simulink model "Hardware_Interface"  (R2021b)
settings: Solver=VariableStepAuto  StartTime=0.0  StopTime=10.0  RelTol=1e-3
settings Model: Creator=Natmatee  LastModifiedBy=Natmatee

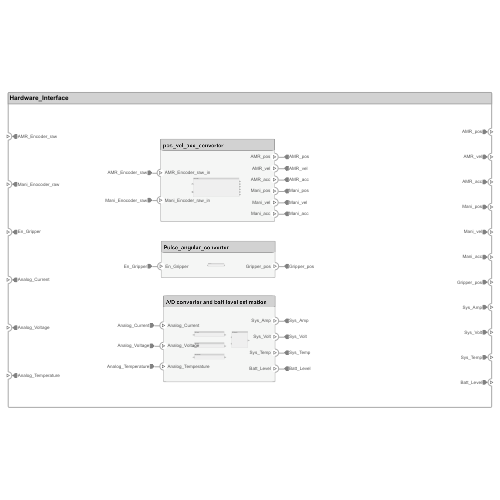
[thumbnail: Simulink's stored preview of the top-level diagram]
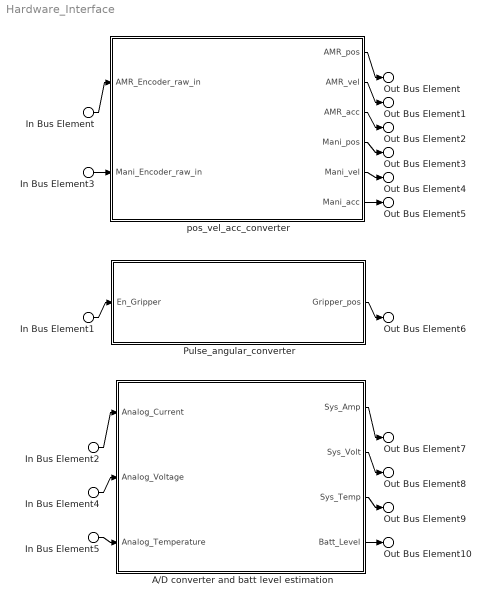
== system Hardware_Interface ==
  In Bus Element : Inport  PortName=AMR_Encoder_raw
  In Bus Element3 : Inport  Port=2  PortName=Mani_Enocoder_raw
  In Bus Element1 : Inport  Port=3  PortName=En_Gripper
  In Bus Element2 : Inport  Port=4  PortName=Analog_Current
  In Bus Element4 : Inport  Port=5  PortName=Analog_Voltage
  In Bus Element5 : Inport  Port=6  PortName=Analog_Temperature
  A/D converter and batt level estimation : Subsystem
      settings: PortSchema="{\"entries\":[{\"content\":{\"headerSize\":26,\"margin\":15,\"minimumSpacing\":25,\"sides\":[{\"content\":{\"connectorIds\":[\"In1\",\"In2\",\"In3\"]},\"type\":\"ConnectorPlacement.EquallySpacedRectSide\",\"uuid\":\"981ec522-52a0-4dbf-ac20-b0bdc6aa1afd\"},{\"content\":{\"connectorIds\":[\"Out1\",\"Out2\",\"Out3\",\"Out4\"],\"side\":\"RIGHT\"},\"type\":\"ConnectorPlacement.EquallySpacedRectSide\",\"uuid\":\"9bffbeba-24b3-4025-8564-8c4b0e924e04\"},{\"content\":{\"connectorIds\":[],\"side\":\"TOP\"},\"type\":\"ConnectorPlacement.EquallySpacedRectSide\",\"uuid\":\"d6517fca-b776-44cd-80b5-050d73676340\"}]},\"type\":\"ConnectorPlacement.EquallySpacedConnector\",\"uuid\":\"152addaa-b2c5-4af4-bfc3-3d7a632ca387\"}],\"packageUris\":[\"http://schema.mathworks.com/mf0/Connector/R2020b\"],\"version\":\"1.0\"}"
  Pulse_angular_converter : Subsystem
      settings: PortSchema="{\"entries\":[{\"content\":{\"headerSize\":26,\"margin\":15,\"minimumSpacing\":25,\"sides\":[{\"content\":{\"connectorIds\":[\"In1\"]},\"type\":\"ConnectorPlacement.EquallySpacedRectSide\",\"uuid\":\"981ec522-52a0-4dbf-ac20-b0bdc6aa1afd\"},{\"content\":{\"connectorIds\":[\"Out1\"],\"side\":\"RIGHT\"},\"type\":\"ConnectorPlacement.EquallySpacedRectSide\",\"uuid\":\"9bffbeba-24b3-4025-8564-8c4b0e924e04\"},{\"content\":{\"connectorIds\":[],\"side\":\"TOP\"},\"type\":\"ConnectorPlacement.EquallySpacedRectSide\",\"uuid\":\"d6517fca-b776-44cd-80b5-050d73676340\"}]},\"type\":\"ConnectorPlacement.EquallySpacedConnector\",\"uuid\":\"152addaa-b2c5-4af4-bfc3-3d7a632ca387\"}],\"packageUris\":[\"http://schema.mathworks.com/mf0/Connector/R2020b\"],\"version\":\"1.0\"}"
  pos_vel_acc_converter : Subsystem
      settings: PortSchema="{\"entries\":[{\"content\":{\"headerSize\":26,\"margin\":15,\"minimumSpacing\":25,\"sides\":[{\"content\":{\"connectorIds\":[\"In1\",\"In2\"]},\"type\":\"ConnectorPlacement.EquallySpacedRectSide\",\"uuid\":\"981ec522-52a0-4dbf-ac20-b0bdc6aa1afd\"},{\"content\":{\"connectorIds\":[\"Out1\",\"Out2\",\"Out3\",\"Out4\",\"Out5\",\"Out6\"],\"side\":\"RIGHT\"},\"type\":\"ConnectorPlacement.EquallySpacedRectSide\",\"uuid\":\"9bffbeba-24b3-4025-8564-8c4b0e924e04\"},{\"content\":{\"connectorIds\":[],\"side\":\"TOP\"},\"type\":\"ConnectorPlacement.EquallySpacedRectSide\",\"uuid\":\"d6517fca-b776-44cd-80b5-050d73676340\"}]},\"type\":\"ConnectorPlacement.EquallySpacedConnector\",\"uuid\":\"152addaa-b2c5-4af4-bfc3-3d7a632ca387\"}],\"packageUris\":[\"http://schema.mathworks.com/mf0/Connector/R2020b\"],\"version\":\"1.0\"}"
  Out Bus Element : Outport  PortName=AMR_pos
  Out Bus Element1 : Outport  Port=2  PortName=AMR_vel
  Out Bus Element2 : Outport  Port=3  PortName=AMR_acc
  Out Bus Element3 : Outport  Port=4  PortName=Mani_pos
  Out Bus Element4 : Outport  Port=5  PortName=Mani_vel
  Out Bus Element5 : Outport  Port=6  PortName=Mani_acc
  Out Bus Element6 : Outport  Port=7  PortName=Gripper_pos
  Out Bus Element7 : Outport  Port=8  PortName=Sys_Amp
  Out Bus Element8 : Outport  Port=9  PortName=Sys_Volt
  Out Bus Element9 : Outport  Port=10  PortName=Sys_Temp
  Out Bus Element10 : Outport  Port=11  PortName=Batt_Level
  wires:
  pos_vel_acc_converter/1(AMR_pos) -> Out Bus Element/1
  pos_vel_acc_converter/2(AMR_vel) -> Out Bus Element1/1
  pos_vel_acc_converter/3(AMR_acc) -> Out Bus Element2/1
  pos_vel_acc_converter/4(Mani_pos) -> Out Bus Element3/1
  pos_vel_acc_converter/5(Mani_vel) -> Out Bus Element4/1
  pos_vel_acc_converter/6(Mani_acc) -> Out Bus Element5/1
  In Bus Element2/1 -> A/D converter and batt level estimation/1(Analog_Current)
  In Bus Element4/1 -> A/D converter and batt level estimation/2(Analog_Voltage)
  In Bus Element5/1 -> A/D converter and batt level estimation/3(Analog_Temperature)
  A/D converter and batt level estimation/1(Sys_Amp) -> Out Bus Element7/1
  A/D converter and batt level estimation/2(Sys_Volt) -> Out Bus Element8/1
  A/D converter and batt level estimation/3(Sys_Temp) -> Out Bus Element9/1
  A/D converter and batt level estimation/4(Batt_Level) -> Out Bus Element10/1
  In Bus Element1/1 -> Pulse_angular_converter/1(En_Gripper)
  Pulse_angular_converter/1(Gripper_pos) -> Out Bus Element6/1
  In Bus Element/1 -> pos_vel_acc_converter/1(AMR_Encoder_raw_in)
  In Bus Element3/1 -> pos_vel_acc_converter/2(Mani_Encoder_raw_in)

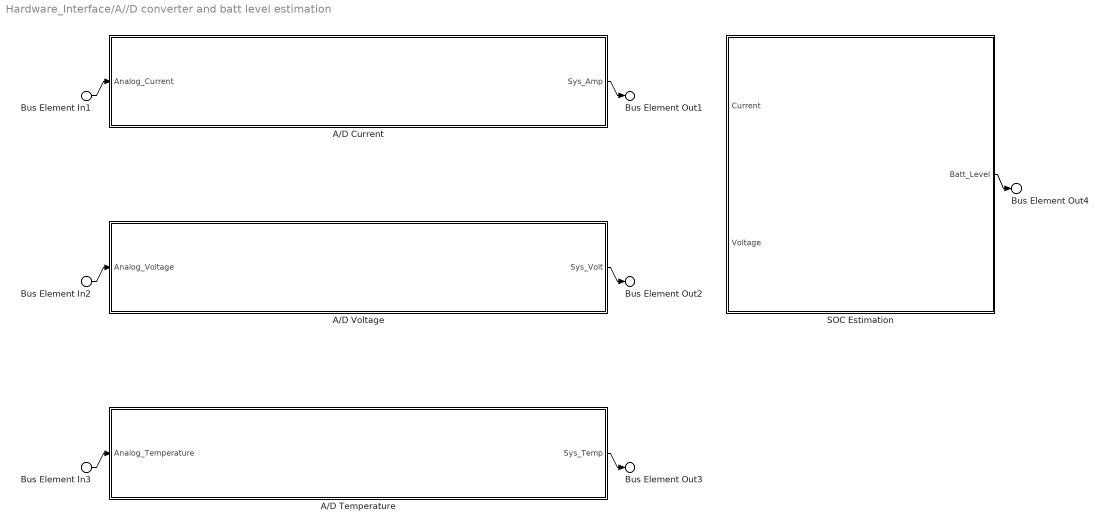
== system Hardware_Interface/A//D converter and batt level estimation ==
  Bus Element In1 : Inport  PortName=Analog_Current
  Bus Element In2 : Inport  Port=2  PortName=Analog_Voltage
  Bus Element In3 : Inport  Port=3  PortName=Analog_Temperature
  A/D Current : Subsystem
      settings: PortSchema="{\"entries\":[{\"content\":{\"headerSize\":26,\"margin\":15,\"minimumSpacing\":25,\"sides\":[{\"content\":{\"connectorIds\":[\"In1\"]},\"type\":\"ConnectorPlacement.EquallySpacedRectSide\",\"uuid\":\"981ec522-52a0-4dbf-ac20-b0bdc6aa1afd\"},{\"content\":{\"connectorIds\":[\"Out1\"],\"side\":\"RIGHT\"},\"type\":\"ConnectorPlacement.EquallySpacedRectSide\",\"uuid\":\"9bffbeba-24b3-4025-8564-8c4b0e924e04\"},{\"content\":{\"connectorIds\":[],\"side\":\"TOP\"},\"type\":\"ConnectorPlacement.EquallySpacedRectSide\",\"uuid\":\"d6517fca-b776-44cd-80b5-050d73676340\"}]},\"type\":\"ConnectorPlacement.EquallySpacedConnector\",\"uuid\":\"152addaa-b2c5-4af4-bfc3-3d7a632ca387\"}],\"packageUris\":[\"http://schema.mathworks.com/mf0/Connector/R2020b\"],\"version\":\"1.0\"}"
  A/D Temperature : Subsystem
      settings: PortSchema="{\"entries\":[{\"content\":{\"headerSize\":26,\"margin\":15,\"minimumSpacing\":25,\"sides\":[{\"content\":{\"connectorIds\":[\"In1\"]},\"type\":\"ConnectorPlacement.EquallySpacedRectSide\",\"uuid\":\"981ec522-52a0-4dbf-ac20-b0bdc6aa1afd\"},{\"content\":{\"connectorIds\":[\"Out1\"],\"side\":\"RIGHT\"},\"type\":\"ConnectorPlacement.EquallySpacedRectSide\",\"uuid\":\"9bffbeba-24b3-4025-8564-8c4b0e924e04\"},{\"content\":{\"connectorIds\":[],\"side\":\"TOP\"},\"type\":\"ConnectorPlacement.EquallySpacedRectSide\",\"uuid\":\"d6517fca-b776-44cd-80b5-050d73676340\"}]},\"type\":\"ConnectorPlacement.EquallySpacedConnector\",\"uuid\":\"152addaa-b2c5-4af4-bfc3-3d7a632ca387\"}],\"packageUris\":[\"http://schema.mathworks.com/mf0/Connector/R2020b\"],\"version\":\"1.0\"}"
  A/D Voltage : Subsystem
      settings: PortSchema="{\"entries\":[{\"content\":{\"headerSize\":26,\"margin\":15,\"minimumSpacing\":25,\"sides\":[{\"content\":{\"connectorIds\":[\"In1\"]},\"type\":\"ConnectorPlacement.EquallySpacedRectSide\",\"uuid\":\"981ec522-52a0-4dbf-ac20-b0bdc6aa1afd\"},{\"content\":{\"connectorIds\":[\"Out1\"],\"side\":\"RIGHT\"},\"type\":\"ConnectorPlacement.EquallySpacedRectSide\",\"uuid\":\"9bffbeba-24b3-4025-8564-8c4b0e924e04\"},{\"content\":{\"connectorIds\":[],\"side\":\"TOP\"},\"type\":\"ConnectorPlacement.EquallySpacedRectSide\",\"uuid\":\"d6517fca-b776-44cd-80b5-050d73676340\"}]},\"type\":\"ConnectorPlacement.EquallySpacedConnector\",\"uuid\":\"152addaa-b2c5-4af4-bfc3-3d7a632ca387\"}],\"packageUris\":[\"http://schema.mathworks.com/mf0/Connector/R2020b\"],\"version\":\"1.0\"}"
  SOC Estimation : Subsystem
      settings: PortSchema="{\"entries\":[{\"content\":{\"headerSize\":26,\"margin\":15,\"minimumSpacing\":25,\"sides\":[{\"content\":{\"connectorIds\":[\"In1\",\"In2\"]},\"type\":\"ConnectorPlacement.EquallySpacedRectSide\",\"uuid\":\"981ec522-52a0-4dbf-ac20-b0bdc6aa1afd\"},{\"content\":{\"connectorIds\":[\"Out1\"],\"side\":\"RIGHT\"},\"type\":\"ConnectorPlacement.EquallySpacedRectSide\",\"uuid\":\"9bffbeba-24b3-4025-8564-8c4b0e924e04\"},{\"content\":{\"connectorIds\":[],\"side\":\"TOP\"},\"type\":\"ConnectorPlacement.EquallySpacedRectSide\",\"uuid\":\"d6517fca-b776-44cd-80b5-050d73676340\"}]},\"type\":\"ConnectorPlacement.EquallySpacedConnector\",\"uuid\":\"152addaa-b2c5-4af4-bfc3-3d7a632ca387\"}],\"packageUris\":[\"http://schema.mathworks.com/mf0/Connector/R2020b\"],\"version\":\"1.0\"}"
  Bus Element Out1 : Outport  PortName=Sys_Amp
  Bus Element Out2 : Outport  Port=2  PortName=Sys_Volt
  Bus Element Out3 : Outport  Port=3  PortName=Sys_Temp
  Bus Element Out4 : Outport  Port=4  PortName=Batt_Level
  wires:
  A/D Current/1(Sys_Amp) -> Bus Element Out1/1
  Bus Element In1/1 -> A/D Current/1(Analog_Current)
  A/D Voltage/1(Sys_Volt) -> Bus Element Out2/1
  Bus Element In2/1 -> A/D Voltage/1(Analog_Voltage)
  Bus Element In3/1 -> A/D Temperature/1(Analog_Temperature)
  A/D Temperature/1(Sys_Temp) -> Bus Element Out3/1
  SOC Estimation/1(Batt_Level) -> Bus Element Out4/1

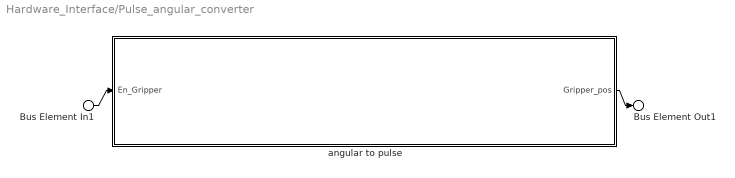
== system Hardware_Interface/Pulse_angular_converter ==
  Bus Element In1 : Inport  PortName=En_Gripper
  angular to pulse : Subsystem
      settings: PortSchema="{\"entries\":[{\"content\":{\"headerSize\":26,\"margin\":15,\"minimumSpacing\":25,\"sides\":[{\"content\":{\"connectorIds\":[\"In1\"]},\"type\":\"ConnectorPlacement.EquallySpacedRectSide\",\"uuid\":\"981ec522-52a0-4dbf-ac20-b0bdc6aa1afd\"},{\"content\":{\"connectorIds\":[\"Out1\"],\"side\":\"RIGHT\"},\"type\":\"ConnectorPlacement.EquallySpacedRectSide\",\"uuid\":\"9bffbeba-24b3-4025-8564-8c4b0e924e04\"},{\"content\":{\"connectorIds\":[],\"side\":\"TOP\"},\"type\":\"ConnectorPlacement.EquallySpacedRectSide\",\"uuid\":\"d6517fca-b776-44cd-80b5-050d73676340\"}]},\"type\":\"ConnectorPlacement.EquallySpacedConnector\",\"uuid\":\"152addaa-b2c5-4af4-bfc3-3d7a632ca387\"}],\"packageUris\":[\"http://schema.mathworks.com/mf0/Connector/R2020b\"],\"version\":\"1.0\"}"
  Bus Element Out1 : Outport  PortName=Gripper_pos
  wires:
  Bus Element In1/1 -> angular to pulse/1(En_Gripper)
  angular to pulse/1(Gripper_pos) -> Bus Element Out1/1

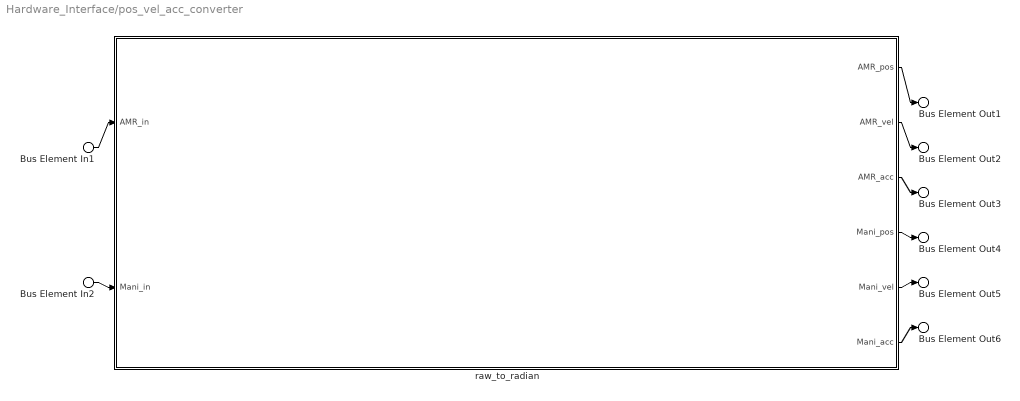
== system Hardware_Interface/pos_vel_acc_converter ==
  Bus Element In1 : Inport  PortName=AMR_Encoder_raw_in
  Bus Element In2 : Inport  Port=2  PortName=Mani_Encoder_raw_in
  raw_to_radian : Subsystem
      settings: PortSchema="{\"entries\":[{\"content\":{\"headerSize\":26,\"margin\":15,\"minimumSpacing\":25,\"sides\":[{\"content\":{\"connectorIds\":[\"In1\",\"In2\"]},\"type\":\"ConnectorPlacement.EquallySpacedRectSide\",\"uuid\":\"981ec522-52a0-4dbf-ac20-b0bdc6aa1afd\"},{\"content\":{\"connectorIds\":[\"Out1\",\"Out2\",\"Out3\",\"Out4\",\"Out5\",\"Out6\"],\"side\":\"RIGHT\"},\"type\":\"ConnectorPlacement.EquallySpacedRectSide\",\"uuid\":\"9bffbeba-24b3-4025-8564-8c4b0e924e04\"},{\"content\":{\"connectorIds\":[],\"side\":\"TOP\"},\"type\":\"ConnectorPlacement.EquallySpacedRectSide\",\"uuid\":\"d6517fca-b776-44cd-80b5-050d73676340\"}]},\"type\":\"ConnectorPlacement.EquallySpacedConnector\",\"uuid\":\"152addaa-b2c5-4af4-bfc3-3d7a632ca387\"}],\"packageUris\":[\"http://schema.mathworks.com/mf0/Connector/R2020b\"],\"version\":\"1.0\"}"
  Bus Element Out1 : Outport  PortName=AMR_pos
  Bus Element Out2 : Outport  Port=2  PortName=AMR_vel
  Bus Element Out3 : Outport  Port=3  PortName=AMR_acc
  Bus Element Out4 : Outport  Port=4  PortName=Mani_pos
  Bus Element Out5 : Outport  Port=5  PortName=Mani_vel
  Bus Element Out6 : Outport  Port=6  PortName=Mani_acc
  wires:
  Bus Element In1/1 -> raw_to_radian/1(AMR_in)
  Bus Element In2/1 -> raw_to_radian/2(Mani_in)
  raw_to_radian/1(AMR_pos) -> Bus Element Out1/1
  raw_to_radian/2(AMR_vel) -> Bus Element Out2/1
  raw_to_radian/3(AMR_acc) -> Bus Element Out3/1
  raw_to_radian/4(Mani_pos) -> Bus Element Out4/1
  raw_to_radian/5(Mani_vel) -> Bus Element Out5/1
  raw_to_radian/6(Mani_acc) -> Bus Element Out6/1

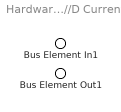
== system Hardware_Interface/A//D converter and batt level estimation/A//D Current ==
  Bus Element In1 : Inport  PortName=Analog_Current
  Bus Element Out1 : Outport  PortName=Sys_Amp

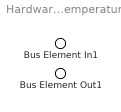
== system Hardware_Interface/A//D converter and batt level estimation/A//D Temperature ==
  Bus Element In1 : Inport  PortName=Analog_Temperature
  Bus Element Out1 : Outport  PortName=Sys_Temp

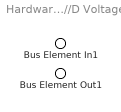
== system Hardware_Interface/A//D converter and batt level estimation/A//D Voltage ==
  Bus Element In1 : Inport  PortName=Analog_Voltage
  Bus Element Out1 : Outport  PortName=Sys_Volt

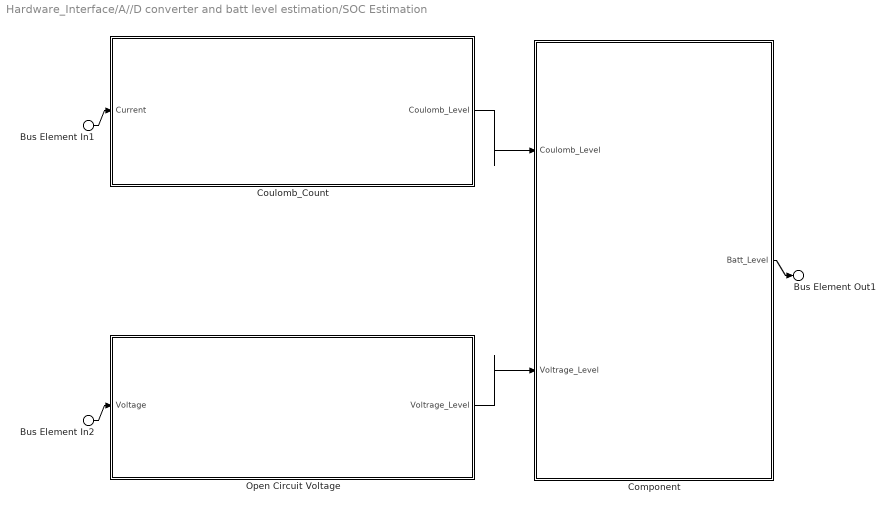
== system Hardware_Interface/A//D converter and batt level estimation/SOC Estimation ==
  Bus Element In1 : Inport  PortName=Current
  Bus Element In2 : Inport  Port=2  PortName=Voltage
  Component : Subsystem
      settings: PortSchema="{\"entries\":[{\"content\":{\"headerSize\":26,\"margin\":15,\"minimumSpacing\":25,\"sides\":[{\"content\":{\"connectorIds\":[\"In1\",\"In2\"]},\"type\":\"ConnectorPlacement.EquallySpacedRectSide\",\"uuid\":\"981ec522-52a0-4dbf-ac20-b0bdc6aa1afd\"},{\"content\":{\"connectorIds\":[\"Out1\"],\"side\":\"RIGHT\"},\"type\":\"ConnectorPlacement.EquallySpacedRectSide\",\"uuid\":\"9bffbeba-24b3-4025-8564-8c4b0e924e04\"},{\"content\":{\"connectorIds\":[],\"side\":\"TOP\"},\"type\":\"ConnectorPlacement.EquallySpacedRectSide\",\"uuid\":\"d6517fca-b776-44cd-80b5-050d73676340\"}]},\"type\":\"ConnectorPlacement.EquallySpacedConnector\",\"uuid\":\"152addaa-b2c5-4af4-bfc3-3d7a632ca387\"}],\"packageUris\":[\"http://schema.mathworks.com/mf0/Connector/R2020b\"],\"version\":\"1.0\"}"
  Coulomb_Count : Subsystem
      settings: PortSchema="{\"entries\":[{\"content\":{\"headerSize\":26,\"margin\":15,\"minimumSpacing\":25,\"sides\":[{\"content\":{\"connectorIds\":[\"In1\"]},\"type\":\"ConnectorPlacement.EquallySpacedRectSide\",\"uuid\":\"981ec522-52a0-4dbf-ac20-b0bdc6aa1afd\"},{\"content\":{\"connectorIds\":[\"Out1\"],\"side\":\"RIGHT\"},\"type\":\"ConnectorPlacement.EquallySpacedRectSide\",\"uuid\":\"9bffbeba-24b3-4025-8564-8c4b0e924e04\"},{\"content\":{\"connectorIds\":[],\"side\":\"TOP\"},\"type\":\"ConnectorPlacement.EquallySpacedRectSide\",\"uuid\":\"d6517fca-b776-44cd-80b5-050d73676340\"}]},\"type\":\"ConnectorPlacement.EquallySpacedConnector\",\"uuid\":\"152addaa-b2c5-4af4-bfc3-3d7a632ca387\"}],\"packageUris\":[\"http://schema.mathworks.com/mf0/Connector/R2020b\"],\"version\":\"1.0\"}"
  Open Circuit Voltage : Subsystem
      settings: PortSchema="{\"entries\":[{\"content\":{\"headerSize\":26,\"margin\":15,\"minimumSpacing\":25,\"sides\":[{\"content\":{\"connectorIds\":[\"In1\"]},\"type\":\"ConnectorPlacement.EquallySpacedRectSide\",\"uuid\":\"981ec522-52a0-4dbf-ac20-b0bdc6aa1afd\"},{\"content\":{\"connectorIds\":[\"Out1\"],\"side\":\"RIGHT\"},\"type\":\"ConnectorPlacement.EquallySpacedRectSide\",\"uuid\":\"9bffbeba-24b3-4025-8564-8c4b0e924e04\"},{\"content\":{\"connectorIds\":[],\"side\":\"TOP\"},\"type\":\"ConnectorPlacement.EquallySpacedRectSide\",\"uuid\":\"d6517fca-b776-44cd-80b5-050d73676340\"}]},\"type\":\"ConnectorPlacement.EquallySpacedConnector\",\"uuid\":\"152addaa-b2c5-4af4-bfc3-3d7a632ca387\"}],\"packageUris\":[\"http://schema.mathworks.com/mf0/Connector/R2020b\"],\"version\":\"1.0\"}"
  Bus Element Out1 : Outport  PortName=Batt_Level
  wires:
  Bus Element In1/1 -> Coulomb_Count/1(Current)
  Bus Element In2/1 -> Open Circuit Voltage/1(Voltage)
  Component/1(Batt_Level) -> Bus Element Out1/1
  Open Circuit Voltage/1(Voltrage_Level) -> Component/2(Voltrage_Level)
  Coulomb_Count/1(Coulomb_Level) -> Component/1(Coulomb_Level)

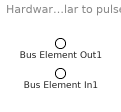
== system Hardware_Interface/Pulse_angular_converter/angular to pulse ==
  Bus Element In1 : Inport  PortName=En_Gripper
  Bus Element Out1 : Outport  PortName=Gripper_pos

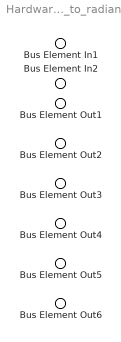
== system Hardware_Interface/pos_vel_acc_converter/raw_to_radian ==
  Bus Element In1 : Inport  PortName=AMR_in
  Bus Element In2 : Inport  Port=2  PortName=Mani_in
  Bus Element Out1 : Outport  PortName=AMR_pos
  Bus Element Out2 : Outport  Port=2  PortName=AMR_vel
  Bus Element Out3 : Outport  Port=3  PortName=AMR_acc
  Bus Element Out4 : Outport  Port=4  PortName=Mani_pos
  Bus Element Out5 : Outport  Port=5  PortName=Mani_vel
  Bus Element Out6 : Outport  Port=6  PortName=Mani_acc

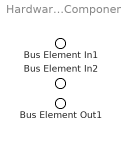
== system Hardware_Interface/A//D converter and batt level estimation/SOC Estimation/Component ==
  Bus Element In1 : Inport  PortName=Coulomb_Level
  Bus Element In2 : Inport  Port=2  PortName=Voltrage_Level
  Bus Element Out1 : Outport  PortName=Batt_Level

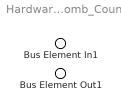
== system Hardware_Interface/A//D converter and batt level estimation/SOC Estimation/Coulomb_Count ==
  Bus Element In1 : Inport  PortName=Current
  Bus Element Out1 : Outport  PortName=Coulomb_Level

== system Hardware_Interface/A//D converter and batt level estimation/SOC Estimation/Open Circuit Voltage ==
  Bus Element In1 : Inport  PortName=Voltage
  Bus Element Out1 : Outport  PortName=Voltrage_Level
